simulink model "peldasensor"  (R2024b)
settings: Solver=VariableStepAuto  StartTime=0.0  StopTime=10.0  RelTol=1e-3
settings Model: Creator=Asus  LastModifiedBy=Asus

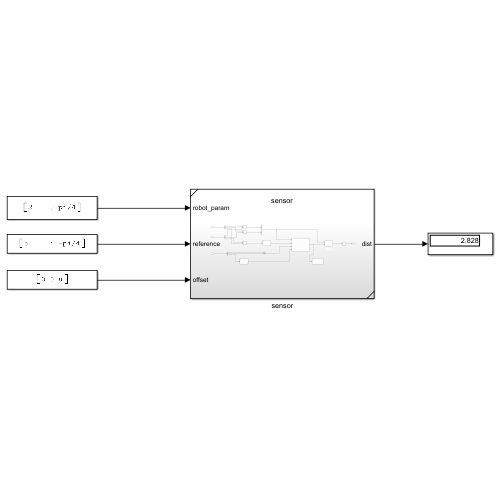
[thumbnail: Simulink's stored preview of the top-level diagram]
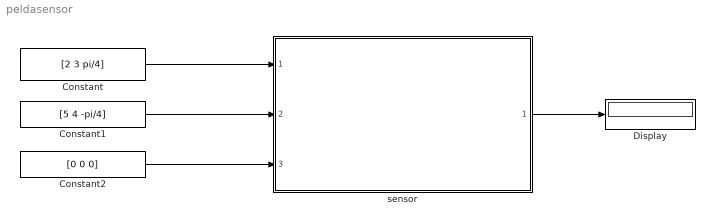
== system peldasensor ==
  Constant : Constant  Value=[2 3 pi/4]
  Constant1 : Constant  Value=[5 4 -pi/4]
  Constant2 : Constant  Value=[0 0 0]
  Display : Display
  sensor : Subsystem  ReferencedSubsystem=sensor
  wires:
  Constant/1 -> sensor/1
  Constant1/1 -> sensor/2
  Constant2/1 -> sensor/3
  sensor/1 -> Display/1
